simulink model "Simulink_Hacheur_P1"  (R2019b)
settings: Solver=ode1  StartTime=0.0  StopTime=0.0001  FixedStep=Ts  RelTol=1e-3
values from neighbouring files (symbols this model uses):
  alpha = 25    [Script_Propulseur_P1.m]
  f = 6.52e-6    (= 6.52e-06)    [Script_Propulseur_P1.m]
  J = (Kem*Kem*tauEm)/Rm    (= 1.1664e-07)    [Script_Propulseur_P1.m]
  Kem = 2.7e-3    (= 0.0027)    [Script_Propulseur_P1.m]
  Lm = 2e-3    (= 0.002)    [Script_Propulseur_P1.m]
  pente = (8.2-6.9)/5    (= 0.26)    [Script_Propulseur_P1.m]
  Rm = 1    [Script_Propulseur_P1.m]
  Te = 5e-5    (= 5e-05)    [Script_Propulseur_P1.m]
libraries: simulink x3
settings Model: Creator=titil  LastModifiedBy=titil

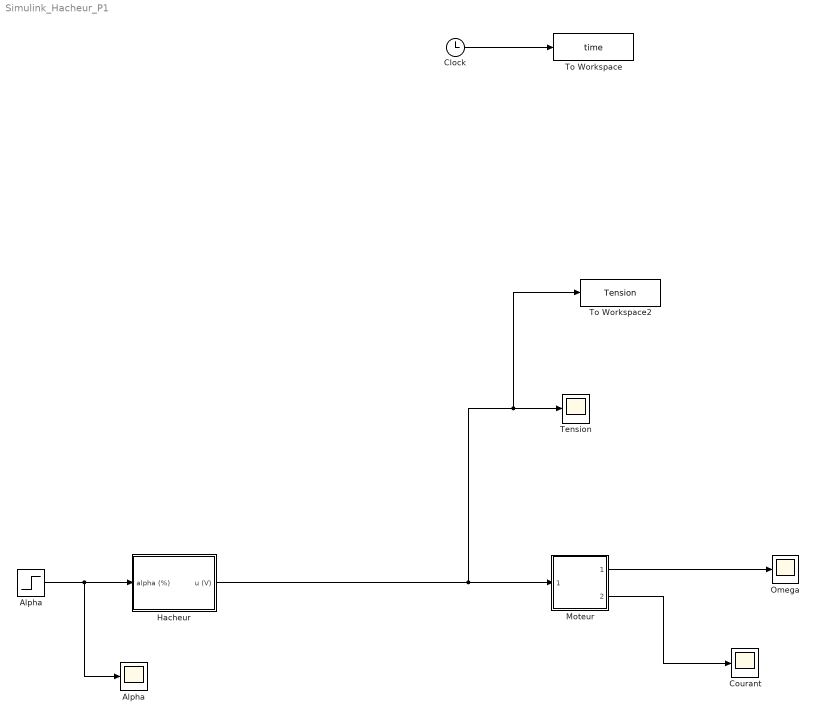
== system Simulink_Hacheur_P1 ==
  Alpha : Step  Time=0  After=alpha  SampleTime=0
  "Alpha " : Scope
  Clock : Clock
  Courant : Scope
  "Hacheur " : Subsystem
  Moteur : Subsystem
  Omega : Scope
  Tension : Scope
  To Workspace : ToWorkspace  VariableName=time  SampleTime=5e-7
      settings: Save2DSignal=2-D array (concatenate along first dimension)
  To Workspace2 : ToWorkspace  VariableName=Tension  SampleTime=5e-7
      settings: Save2DSignal=2-D array (concatenate along first dimension)
  wires:
  Alpha/1 -> "Alpha "/1, "Hacheur "/1(alpha (%))
  Moteur/2(Omega) -> Courant/1
  "Hacheur "/1(u (V)) -> Moteur/1(Tension), To Workspace2/1, Tension/1
  Moteur/1(Courant) -> Omega/1
  Clock/1 -> To Workspace/1

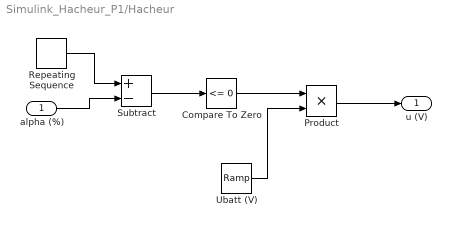
== system Simulink_Hacheur_P1/Hacheur  ==
  alpha (%) : Inport
  Compare To Zero : simulink/Logic and Bit Operations/Compare To Zero  relop=<=  OutDataTypeStr=boolean
  Product : Product
  Repeating Sequence : simulink/Sources/Repeating Sequence  rep_seq_t=[0 Te]  rep_seq_y=[1 100]
  Subtract : Sum  Inputs=+-
  Ubatt (V) : simulink/Sources/Ramp  slope=-pente  start=0  InitialOutput=8.2
  u (V) : Outport
  wires:
  Subtract/1 -> Compare To Zero/1
  Ubatt (V)/1 -> Product/2
  Product/1 -> u (V)/1
  Compare To Zero/1 -> Product/1
  Repeating Sequence/1 -> Subtract/1
  alpha (%)/1 -> Subtract/2

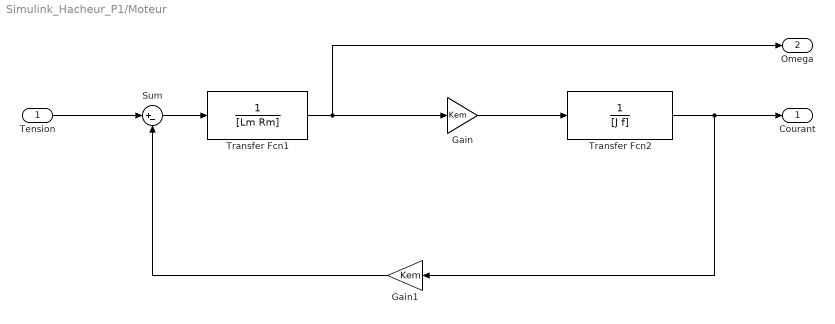
== system Simulink_Hacheur_P1/Moteur ==
  Tension : Inport
  Gain : Gain  Gain=Kem
  Gain1 : Gain  Gain=Kem
  Sum : Sum  Inputs=|+-
  Transfer Fcn1 : TransferFcn  Denominator=[Lm Rm]
  Transfer Fcn2 : TransferFcn  Denominator=[J f]
  Courant : Outport
  Omega : Outport  Port=2
  wires:
  Sum/1 -> Transfer Fcn1/1
  Gain1/1 -> Sum/2
  Transfer Fcn2/1 -> Courant/1, Gain1/1
  Transfer Fcn1/1 -> Omega/1, Gain/1
  Gain/1 -> Transfer Fcn2/1
  Tension/1 -> Sum/1
